simulink model "malthus"  (R2023b)
settings: Solver=VariableStepAuto  StartTime=0.0  StopTime=10  RelTol=1e-3
values from neighbouring files (symbols this model uses):
  N0 = 100    [dinamica_popolazioni.m]
settings Model: Creator=stefa  LastModifiedBy=stefa

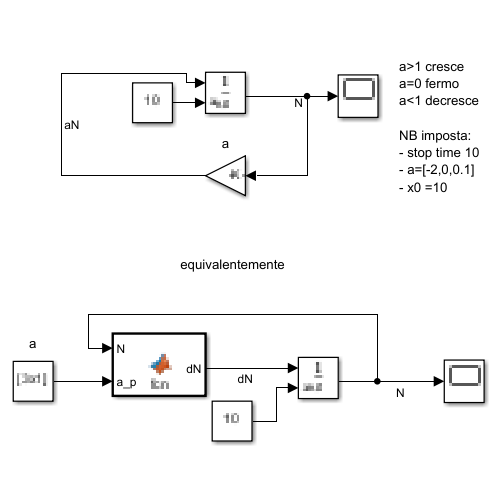
[thumbnail: Simulink's stored preview of the top-level diagram]
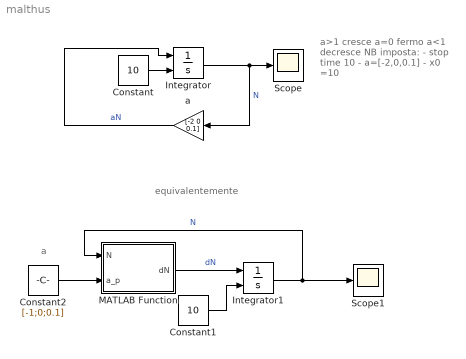
== system malthus ==
  note: a
  note: equivalentemente
  note: a>1 cresce
      | a=0 fermo
      | a<1 decresce
      |
      | NB imposta:
      | - stop time 10
      | - a=[-2,0,0.1]
      | - x0 =10
  Constant : Constant  Value=10
  Constant1 : Constant  Value=10
  Constant2 : Constant  Value=[-1;0;0.1]
  Integrator : Integrator  InitialConditionSource=external  InitialCondition=N0
  Integrator1 : Integrator  InitialConditionSource=external
  MATLAB Function : MATLAB Function  TreatAsAtomicUnit=on
  Scope : Scope
  Scope1 : Scope
  a : Gain  Gain=[-2 0 0.1]
  wires:
  Integrator/1 -> a/1, Scope/1  "N"
  a/1 -> Integrator/1  "aN"
  Constant/1 -> Integrator/2
  MATLAB Function/1(dN) -> Integrator1/1  "dN"
  Integrator1/1 -> MATLAB Function/1(N), Scope1/1  "N"
  Constant1/1 -> Integrator1/2
  Constant2/1 -> MATLAB Function/2(a_p)

== matlab function malthus/MATLAB Function ==
  data: N input; dN output; a_p input
function dN = fcn(N,a_p)

dN= a_p.*N;
